simulink model "outputs"  (R2020a)
settings: Solver=VariableStepAuto  StartTime=0.0  StopTime=20  RelTol=1e-3
values from neighbouring files (symbols this model uses):
  dry_mass_N = dry_mass*4.44822    (= 27.2675886)    [engineMassModelM.m]
  isp_gain = 0.04376923077    [engineMassModelM.m]
  isp_offset = 2705.153846    [engineMassModelM.m]
settings Model: Creator=Makar  LastModifiedBy=Makar

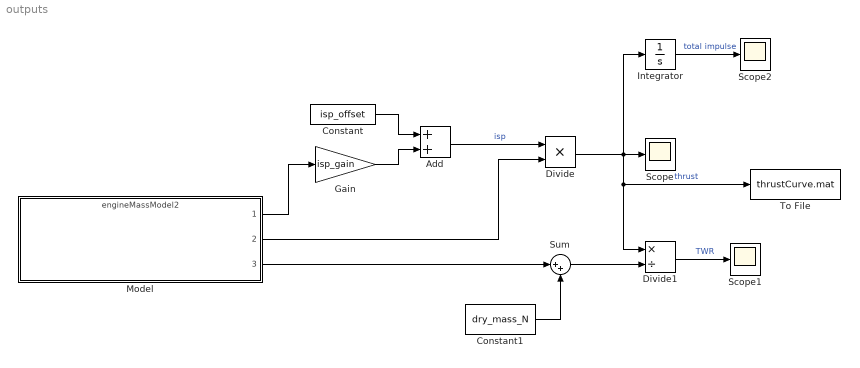
== system outputs ==
  Add : Sum
  Constant : Constant  Value=isp_offset
  Constant1 : Constant  Value=dry_mass_N
  Divide : Product  Inputs=**
  Divide1 : Product  Inputs=*/
  Gain : Gain  Gain=isp_gain
  Integrator : Integrator
  Model : ModelReference  ModelNameDialog=engineMassModel2.slx  SimulationMode=Normal  ModelReferenceVersion=1.5
  Scope : Scope
  Scope1 : Scope
  Scope2 : Scope
  Sum : Sum  Inputs=|++
  To File : ToFile  Filename=thrustCurve.mat  MatrixName=thrust
  wires:
  Gain/1 -> Add/2
  Constant/1 -> Add/1
  Model/1 -> Gain/1
  Add/1 -> Divide/1  "isp"
  Model/2 -> Divide/2
  Divide/1 -> Integrator/1, To File/1, Divide1/1, Scope/1  "thrust"
  Model/3 -> Sum/1
  Constant1/1 -> Sum/2
  Sum/1 -> Divide1/2
  Divide1/1 -> Scope1/1  "TWR"
  Integrator/1 -> Scope2/1  "total impulse"
